simulink model "Aerosonde_simulation_model"  (R2020b)
settings: Solver=ode45  StartTime=0.0  StopTime=1000  RelTol=1e-6
libraries: simulink_extras x3, shared6dof x1, aerolibatmos2 x1, aerolibanimutils x1, etargetslib x1, dspnetwork x1
settings Model: SimulationMode=accelerator  EnablePacing=on  Creator=Cheng  LastModifiedBy=Cheng

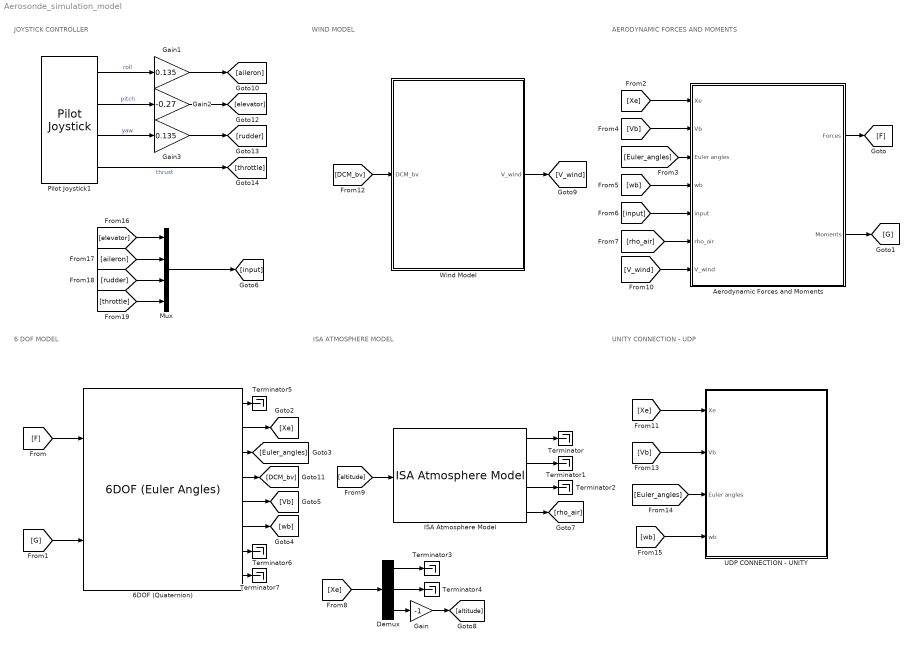
== system Aerosonde_simulation_model ==
  note: UNITY CONNECTION - UDP
  note: ISA ATMOSPHERE MODEL
  note: WIND MODEL
  note: JOYSTICK CONTROLLER
  note: AERODYNAMIC FORCES AND MOMENTS
  note: 6 DOF MODEL
  6DOF (Quaternion) : shared6dof/6DOF (Euler Angles)  units=Metric (MKS)  mtype=Fixed  rep=Quaternion  xme_0=[2100 2300 -200]  Vm_0=[25 0 0]  eul_0=[0 0 4.71]  pm_0=[0 0 0]  mass_0=11.0  mass_e=0.5  mass_f=2.0  inertia=[0.824 0 0; 0 1.135 0; 0 0 1.759]  inertia_e=eye(3)  inertia_f=2*eye(3)  k_quat=1  vre_flag=on  abi_flag=off  aMode=0  xme_statename=''  Vm_statename=''  eul_statename=''  quat_statename=''  pm_statename=''  mass_statename=''
      settings: SourceProductBaseCode=AE,PW,MT,UV,VE,VP
  Aerodynamic Forces and Moments : Subsystem
  Demux : Demux  Outputs=3
  Gain : Gain  Gain=-1
  Gain1 : Gain  Gain=0.135
  Gain2 : Gain  Gain=-0.27
  Gain3 : Gain  Gain=0.135
  ISA Atmosphere Model : aerolibatmos2/ISA Atmosphere Model  custom=off  g=9.80665  gamma=1.4  R=287.0531  L=0.0065  h_trop=11000  h_strat=20000  rho0=1.225  P0=101325  T0=288.15  h0=0
  Mux : Mux
  Pilot Joystick1 : aerolibanimutils/Pilot Joystick  JoystickID=Joystick1  OutputConfiguration=FourAxis  SampleTime=1/30
  Terminator{,1..7} (8 alike) : Terminator
  UDP CONNECTION - UNITY : Subsystem
  Wind Model : Subsystem  mask{wind_n=0, wind_e=0, wind_d=0, L_u=200, L_v=200, L_w=50, sigma_u=1.06, sigma_v=1.06, sigma_w=0.7, Va_0=0}
      mask prompts: wind_n "North Compenent of Wind (wind_n)"; wind_e "East Compenent of Wind (wind_e)"; wind_d "Down Compenent of Wind (wind_d)"; L_u "x Component of Spatial Wavelength (L_u)"; L_v "y Component of Spatial Wavelength (L_v)"; L_w "z Component of Spatial Wavelength (L_w)"; sigma_u "x Component of Intensity (sigma_u)"; sigma_v "y Component of Intensity (sigma_v)"; sigma_w "z Component of Intensity (sigma_w)"; Va_0 "Initial Value of Airspeed"
      mask DialogControl Container4 Prompt: Wind Constants
  wires:
  Demux/3 -> Gain/1
  6DOF (Quaternion)/4 -> [DCM_bv]
  Aerodynamic Forces and Moments/1("Forces ") -> [F]
  [altitude] -> ISA Atmosphere Model/1
  6DOF (Quaternion)/7 -> Terminator6/1
  [rho_air] -> Aerodynamic Forces and Moments/6(rho_air)
  Demux/2 -> Terminator4/1
  Wind Model/1(V_wind) -> [V_wind]
  Aerodynamic Forces and Moments/2(Moments) -> [G]
  [V_wind] -> Aerodynamic Forces and Moments/7(V_wind)
  Demux/1 -> Terminator3/1
  [DCM_bv] -> Wind Model/1(DCM_bv)
  [Euler_angles] -> Aerodynamic Forces and Moments/3(Euler angles)
  6DOF (Quaternion)/1 -> Terminator5/1
  6DOF (Quaternion)/5 -> [Vb]
  [input] -> Aerodynamic Forces and Moments/5(input)
  [G] -> 6DOF (Quaternion)/2
  [Xe] -> Aerodynamic Forces and Moments/1(Xe)
  [Xe] -> Demux/1
  [F] -> 6DOF (Quaternion)/1
  [wb] -> Aerodynamic Forces and Moments/4(wb)
  6DOF (Quaternion)/6 -> [wb]
  6DOF (Quaternion)/3 -> [Euler_angles]
  ISA Atmosphere Model/4 -> [rho_air]
  6DOF (Quaternion)/2 -> [Xe]
  Gain/1 -> [altitude]
  ISA Atmosphere Model/2 -> Terminator1/1
  ISA Atmosphere Model/3 -> Terminator2/1
  6DOF (Quaternion)/8 -> Terminator7/1
  ISA Atmosphere Model/1 -> Terminator/1
  [Vb] -> Aerodynamic Forces and Moments/2(Vb)
  [Xe] -> UDP CONNECTION - UNITY/1(Xe)
  [Vb] -> UDP CONNECTION - UNITY/2(Vb)
  [Euler_angles] -> UDP CONNECTION - UNITY/3(Euler angles)
  [wb] -> UDP CONNECTION - UNITY/4(wb)
  Gain1/1 -> [aileron]
  Gain2/1 -> [elevator]
  Gain3/1 -> [rudder]
  Pilot Joystick1/4 -> [throttle]  "thrust"
  Pilot Joystick1/2 -> Gain2/1  "pitch"
  Pilot Joystick1/3 -> Gain3/1  "yaw"
  Pilot Joystick1/1 -> Gain1/1  "roll"
  [elevator] -> Mux/1
  [aileron] -> Mux/2
  [rudder] -> Mux/3
  [throttle] -> Mux/4
  Mux/1 -> [input]

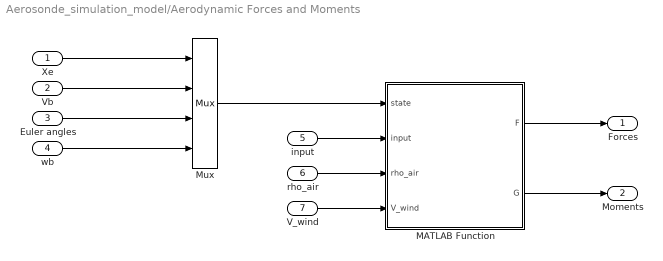
== system Aerosonde_simulation_model/Aerodynamic Forces and Moments ==
  Xe : Inport
  Vb : Inport  Port=2
  Euler angles : Inport  Port=3
  wb : Inport  Port=4
  input : Inport  Port=5
  rho_air : Inport  Port=6
  V_wind : Inport  Port=7
  MATLAB Function : MATLAB Function  TreatAsAtomicUnit=on
  Mux : Mux
  "Forces " : Outport
  Moments : Outport  Port=2
  wires:
  Euler angles/1 -> Mux/3
  wb/1 -> Mux/4
  Mux/1 -> MATLAB Function/1(state)
  Vb/1 -> Mux/2
  Xe/1 -> Mux/1
  MATLAB Function/1(F) -> "Forces "/1
  MATLAB Function/2(G) -> Moments/1
  input/1 -> MATLAB Function/2(input)
  rho_air/1 -> MATLAB Function/3(rho_air)
  V_wind/1 -> MATLAB Function/4(V_wind)

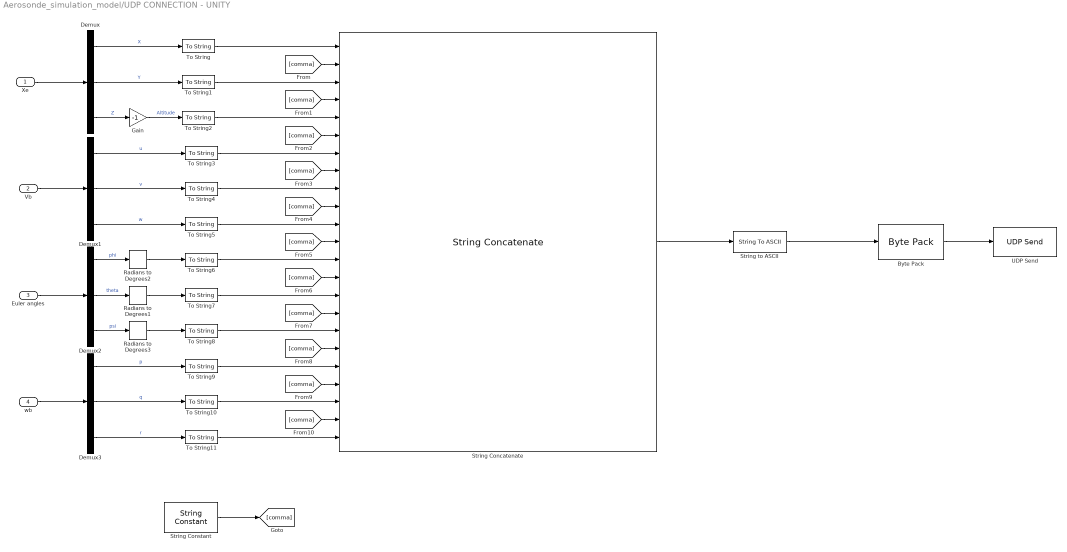
== system Aerosonde_simulation_model/UDP CONNECTION - UNITY ==
  Xe : Inport
  Vb : Inport  Port=2
  Euler angles : Inport  Port=3
  wb : Inport  Port=4
  Byte Pack : etargetslib/Byte Pack  datatypes={'uint8'}  byteAlign=1
  Demux{,1..3} (4 alike) : Demux  Outputs=3
  Gain : Gain  Gain=-1
  Radians to Degrees1 : simulink_extras/Transformations/Radians to Degrees
  Radians to Degrees2 : simulink_extras/Transformations/Radians to Degrees
  Radians to Degrees3 : simulink_extras/Transformations/Radians to Degrees
  String Concatenate : StringConcatenate  Inputs=23
  String Constant : StringConstant  String="\",\""
  String to ASCII : StringToASCII  OutputVectorSize=128
  To String{,1..11} (12 alike) : ToString
  UDP Send : dspnetwork/UDP Send  remoteURL='127.0.0.1'  remotePort=1234  localURL='0.0.0.0'  localPortSource=Automatically determine  localPort=-1  sendBufferSize=8192  sampletime=-1  blockPlatform=[]  separateLengthPort=0
  wires:
  Xe/1 -> Demux/1
  Vb/1 -> Demux1/1
  Euler angles/1 -> Demux2/1
  wb/1 -> Demux3/1
  Demux/2 -> To String1/1  "Y"
  Demux/3 -> Gain/1  "Z"
  Demux1/1 -> To String3/1  "u"
  Demux1/2 -> To String4/1  "v"
  Demux1/3 -> To String5/1  "w"
  Demux2/1 -> Radians to Degrees2/1  "phi"
  Demux2/2 -> Radians to Degrees1/1  "theta"
  Demux2/3 -> Radians to Degrees3/1  "psi"
  Demux3/1 -> To String9/1  "p"
  Demux3/2 -> To String10/1  "q"
  Demux3/3 -> To String11/1  "r"
  String Constant/1 -> [comma]
  [comma] -> String Concatenate/2
  [comma] -> String Concatenate/4
  [comma] -> String Concatenate/6
  [comma] -> String Concatenate/8
  [comma] -> String Concatenate/10
  [comma] -> String Concatenate/12
  [comma] -> String Concatenate/14
  [comma] -> String Concatenate/16
  [comma] -> String Concatenate/18
  [comma] -> String Concatenate/20
  [comma] -> String Concatenate/22
  To String/1 -> String Concatenate/1
  To String1/1 -> String Concatenate/3
  To String2/1 -> String Concatenate/5
  To String3/1 -> String Concatenate/7
  To String4/1 -> String Concatenate/9
  To String5/1 -> String Concatenate/11
  To String6/1 -> String Concatenate/13
  To String7/1 -> String Concatenate/15
  To String8/1 -> String Concatenate/17
  To String9/1 -> String Concatenate/19
  To String10/1 -> String Concatenate/21
  To String11/1 -> String Concatenate/23
  String Concatenate/1 -> String to ASCII/1
  String to ASCII/1 -> Byte Pack/1
  Byte Pack/1 -> UDP Send/1
  Radians to Degrees1/1 -> To String7/1
  Demux/1 -> To String/1  "X"
  Radians to Degrees2/1 -> To String6/1
  Radians to Degrees3/1 -> To String8/1
  Gain/1 -> To String2/1  "Altitude"

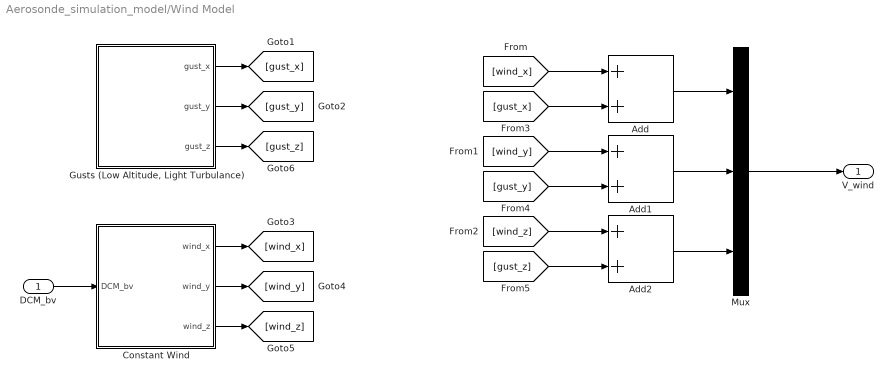
== system Aerosonde_simulation_model/Wind Model ==
  DCM_bv : Inport
  Add : Sum
  Add1 : Sum
  Add2 : Sum
  "Constant Wind " : Subsystem
  "Gusts (Low Altitude, Light Turbulance)" : Subsystem
  Mux : Mux  Inputs=3
  V_wind : Outport
  wires:
  Mux/1 -> V_wind/1
  DCM_bv/1 -> "Constant Wind "/1(DCM_bv)
  "Constant Wind "/1(wind_x) -> [wind_x]
  "Constant Wind "/2(wind_y) -> [wind_y]
  "Constant Wind "/3(wind_z) -> [wind_z]
  Add/1 -> Mux/1
  Add1/1 -> Mux/2
  Add2/1 -> Mux/3
  [wind_y] -> Add1/1
  [wind_x] -> Add/1
  [wind_z] -> Add2/1
  "Gusts (Low Altitude, Light Turbulance)"/3(gust_z) -> [gust_z]
  "Gusts (Low Altitude, Light Turbulance)"/2(gust_y) -> [gust_y]
  "Gusts (Low Altitude, Light Turbulance)"/1(gust_x) -> [gust_x]
  [gust_x] -> Add/2
  [gust_y] -> Add1/2
  [gust_z] -> Add2/2

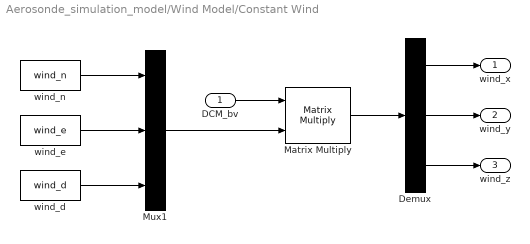
== system Aerosonde_simulation_model/Wind Model/Constant Wind  ==
  DCM_bv : Inport
  Demux : Demux  Outputs=3
  Matrix Multiply : Product  Multiplication=Matrix(*)
  Mux1 : Mux  Inputs=3
  wind_d : Constant  Value=wind_d
  wind_e : Constant  Value=wind_e
  wind_n : Constant  Value=wind_n
  wind_x : Outport
  wind_y : Outport  Port=2
  wind_z : Outport  Port=3
  wires:
  Demux/1 -> wind_x/1
  Matrix Multiply/1 -> Demux/1
  DCM_bv/1 -> Matrix Multiply/1
  Demux/2 -> wind_y/1
  Mux1/1 -> Matrix Multiply/2
  wind_d/1 -> Mux1/3
  wind_n/1 -> Mux1/1
  wind_e/1 -> Mux1/2
  Demux/3 -> wind_z/1

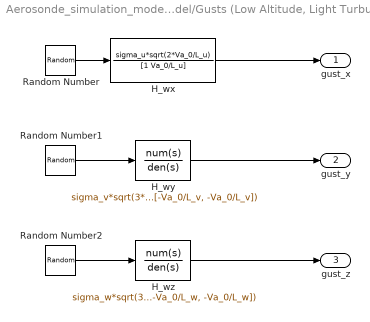
== system Aerosonde_simulation_model/Wind Model/Gusts (Low Altitude, Light Turbulance) ==
  H_wx : TransferFcn  Numerator=sigma_u*sqrt(2*Va_0/L_u)  Denominator=[1 Va_0/L_u]
  H_wy : TransferFcn  Numerator=sigma_v*sqrt(3*Va_0/L_v)*[0, 1,Va_0/sqrt(3)/L_v]  Denominator=poly([-Va_0/L_v, -Va_0/L_v])
  H_wz : TransferFcn  Numerator=sigma_w*sqrt(3*Va_0/L_w)*[0, 1,Va_0/sqrt(3)/L_w]  Denominator=poly([-Va_0/L_w, -Va_0/L_w])
  Random Number : RandomNumber  SampleTime=0
  Random Number1 : RandomNumber  SampleTime=0
  Random Number2 : RandomNumber  SampleTime=0
  gust_x : Outport
  gust_y : Outport  Port=2
  gust_z : Outport  Port=3
  wires:
  H_wy/1 -> gust_y/1
  Random Number2/1 -> H_wz/1
  Random Number/1 -> H_wx/1
  H_wz/1 -> gust_z/1
  Random Number1/1 -> H_wy/1
  H_wx/1 -> gust_x/1

== matlab function Aerosonde_simulation_model/Aerodynamic Forces and Moments/MATLAB Function ==
  data: state input; F output; G output; input input; rho_air input; V_wind input
function [F,G] = fcn(state,input,rho_air,V_wind)

% ************************* States of the aircraft ***********************

%Position with respect to Inertial frame
%It is written in the NED coordinate system
    
pn      = state(1);
pe      = state(2);
pd      = state(3);
%Velocity in the body fixed coordinate system
    
u       = state(4);
v       = state(5);
w       = state(6); 

%Euler angles
phi      = state(7);            
theta    = state(8);       
psi      = state(9); 

%Angular rates in the body fixed coordinate system
p       = state(10);
q       = state(11);
r       = state(12);

 % ************************* Inputs of the aircraft ***********************
 delta_e = input(1);
 delta_a = input(2);
 delta_r = input(3);
 delta_t = input(4);
 
 % ************************* Wind Parameters ***********************
 u_wind = V_wind(1);
 v_wind = V_wind(2);
 w_wind = V_wind(3);
 
 u_r = u - u_wind;
 v_r = v - v_wind;
 w_r = w - w_wind;
 
 Va = norm([u_r v_r w_r]); %Airspeed
 alpha = atan(w_r/u_r); % Angle of attack
 beta = asin(v_r/Va); % Side-slip angle

% ***********************PHYSICAL PARAMETERS OF AIRCRAFT*********************
mav_mass = 11.0;
mav_gravity = 9.81;
mav_Jx   = 0.824;
mav_Jy   = 1.135;
mav_Jz   = 1.759;
mav_Jxz  = 0.120;

% ************************AERODYNAMICS COEFFICIENTS**************************
mav_S_wing        = 0.55;   % Area
mav_b             = 2.90;   % Wingspan
mav_c             = 0.19;   % Chord
mav_S_prop        = 0.2027;
mav_rho           = rho_air;
mav_k_motor       = 80;
mav_k_T_P         = 0;     % No torque
mav_k_Omega       = 0;     % No torque
mav_e             = 0.9;
mav_AR            = mav_b^2/mav_S_wing;


mav_C_L_0         = 0.23;
mav_C_L_alpha     = 5.61;
mav_C_L_q         = 7.95;
mav_C_L_delta_e   = 0.13;
%--------
mav_C_D_0         = 0.043;
mav_C_D_alpha     = 0.030;
mav_C_D_p         = 0.0;
mav_C_D_q         = 0.0;
mav_C_D_delta_e   = 0.0135;
%--------
mav_C_m_0         = 0.0135;
mav_C_m_alpha     = -2.71;           % Longitudinal static stability derivative
mav_C_m_q         = -38.2;           % Pitch damping derivative
mav_C_m_delta_e   = -0.99;           % Primary control derivative
%--------
mav_C_Y_0         = 0.0;             % For symmetric aircraft
mav_C_Y_beta      = -0.83;
mav_C_Y_p         = 0.0;
mav_C_Y_r         = 0.0;
mav_C_Y_delta_a   = 0.075;
mav_C_Y_delta_r   = 0.19;
%--------
mav_C_ell_0       = 0.0;             % For symmetric aircraft
mav_C_ell_beta    = -0.13;           % Roll static stability derivative  -0.13
mav_C_ell_p       = -0.51;           % Roll damping derivative           -0.51
mav_C_ell_r       = 0.045;
mav_C_ell_delta_a = 0.17;            % Primary control derivative
mav_C_ell_delta_r = 0.0024;          % Cross-control derivative
%--------
mav_C_n_0         = 0.0;             % For symmetric aircraft
mav_C_n_beta      = 0.073;           % Yaw static stability derivative   0.073
mav_C_n_p         = -0.069;
mav_C_n_r         = -0.155;          % Yaw damping derivative            -0.095
mav_C_n_delta_a   = -0.011;          % Cross-control derivative
mav_C_n_delta_r   = -0.069;          % Primary control derivative
mav_C_prop        = 1.0;
%     % HACK: prop has too much power for aerosonde
%     mav_C_prop = 0.5;
mav_M             = 50;
mav_epsilon       = 0.16;
mav_alpha0        = 0.47;


% ***************************PROP PARAMETERS********************************* 
mav_D_prop = 20*(0.0254);     % prop diameter in m


% ****************************MOTOR PARAMETERS*******************************
mav_K_V = 145;                    % from datasheet RPM/V
mav_KQ = (1/mav_K_V)*60/(2*pi);   % KQ in N-m/A, V-s/rad
mav_R_motor = 0.042;              % ohms
mav_i0 = 1.5;                     % no-load (zero-torque) current (A)

% Inputs
mav_ncells = 12;
mav_V_max = 3.7*mav_ncells;       % max voltage for specified number of battery cells

% Coeffiecients from prop_data fit
mav_C_Q2 = -0.01664;
mav_C_Q1 = 0.004970;
mav_C_Q0 = 0.005230;

mav_C_T2 = -0.1079;
mav_C_T1 = -0.06044;
mav_C_T0 = 0.09357;

% **************************** CALCULATION *******************************
%Aerodynamic Coefficients
sigma = (1+exp(-mav_M*(alpha-mav_alpha0))+exp(mav_M*(alpha+mav_alpha0)))/...
        ((1+exp(-mav_M*(alpha-mav_alpha0)))*(1+exp(mav_M*(alpha+mav_alpha0))));
Cl = (1-sigma)*(mav_C_L_0+mav_C_L_alpha*alpha) + ...
       sigma*(2*sign(alpha)*sin(alpha)^2*cos(alpha));
Cd = mav_C_D_0 + ((mav_C_L_0+mav_C_L_alpha*alpha)^2)/(pi*mav_e*mav_b^2/mav_S_wing);
Cx = -Cd*cos(alpha)+Cl*sin(alpha);
Cx_q = -mav_C_D_q*cos(alpha)+mav_C_L_q*sin(alpha);
Cx_delta_e = -mav_C_D_delta_e*cos(alpha)+mav_C_L_delta_e*sin(alpha);
Cz = -Cd*sin(alpha)-Cl*cos(alpha);
Cz_q = -mav_C_D_q*sin(alpha)-mav_C_L_q*cos(alpha);
Cz_delta_e = -mav_C_D_delta_e*sin(alpha)-mav_C_L_delta_e*cos(alpha);

%Forces
F = [-mav_mass*mav_gravity*sin(theta) + ...
          0.5*mav_rho*(Va^2)*mav_S_wing * (Cx + Cx_q*(mav_c/(2*Va))*q + Cx_delta_e*delta_e) + ...
          0.5*mav_rho*mav_S_prop*mav_C_prop * ((mav_k_motor*delta_t)^2-Va^2);...
                
           mav_mass*mav_gravity*cos(theta)*sin(phi) + ...
           0.5*mav_rho*(Va^2)*mav_S_wing * (mav_C_Y_0 + mav_C_Y_beta*beta + mav_C_Y_p*(mav_b/(2*Va))*p + ...
           mav_C_Y_r*(mav_b/(2*Va))*r + mav_C_Y_delta_a*delta_a + mav_C_Y_delta_r*delta_r);...
           
           mav_mass*mav_gravity*cos(theta)*cos(phi) + ...
           0.5*mav_rho*(Va^2)*mav_S_wing * (Cz + Cz_q*(mav_c/(2*Va))*q + Cz_delta_e*delta_e)];
                

%Moments
G = [0.5*mav_rho*(Va^2)*mav_S_wing * mav_b * ...
    (mav_C_ell_0 + mav_C_ell_beta*beta + mav_C_ell_p*(mav_b/(2*Va))*p + mav_C_ell_r*(mav_b/(2*Va))*r +...
     mav_C_ell_delta_a*delta_a + mav_C_ell_delta_r*delta_r) - ...
     mav_k_T_P*((mav_k_Omega*delta_t)^2); ...
     
     0.5*mav_rho*(Va^2)*mav_S_wing * mav_c * ...
     (mav_C_m_0 + mav_C_m_alpha*alpha + mav_C_m_q*(mav_c/(2*Va))*q + mav_C_m_delta_e*delta_e);...
     
     0.5*mav_rho*(Va^2)*mav_S_wing * mav_b * ...
        (mav_C_n_0 + mav_C_n_beta*beta + mav_C_n_p*(mav_b/(2*Va))*p + mav_C_n_r*(mav_b/(2*Va))*r + ...
         mav_C_n_delta_a*delta_a + mav_C_n_delta_r*delta_r)];
end
